simulink model "rocket_model"  (R2012b)
settings: Solver=ode3  StartTime=0.0  StopTime=100  MaxStep=.01  RelTol=1e-3
values from neighbouring files (symbols this model uses):
  coef_body = [0; 0; 0; 0; 0; 0]    [rocket_model_matlab.m]
  cp = [1.2; 0; 0]    [rocket_model_matlab.m]
  dyear = decyear('13-January-2014','dd-mmm-yyyy')    [rocket_model_matlab.m]
  href = 0    [rocket_model_matlab.m]
  lat = 37.4292    [rocket_model_matlab.m]
  lon = -122.1381    [rocket_model_matlab.m]
  phi0 = .1    (= 0.1)    [rocket_model_matlab.m]
  psi0 = -0.3    [rocket_model_matlab.m]
  theta0 = pi/2+.2    (= 1.77079632679)    [rocket_model_matlab.m]
  threshold = 0    [rocket_model_matlab.m]
  Thruster_Moment = r*Thruster_Thrust    (= 0.05)    [rocket_model_matlab.m]
  Thruster_Thrust = 1    [rocket_model_matlab.m]
undefined symbols (not defined in the file or in its folder): Earth, WGS84
libraries: aerolibgravity2 x2, aerolibtransform2 x2, aerolibbdyn x2, aerolibutil x2, aerolibanim x1, aerolibadyn x1, aerolibasang x1, aerolibatmos2 x1, aerolib6dof2 x1, simulink x1
settings Model: Creator=Robbie  LastModifiedBy=Robbie

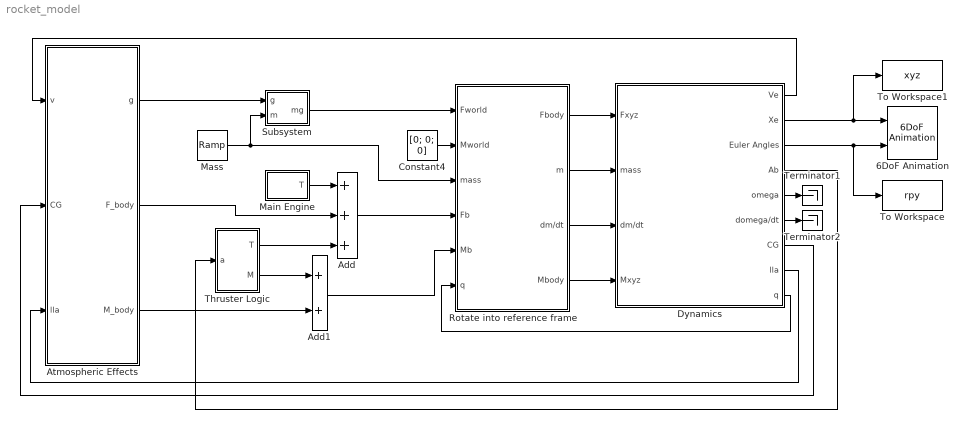
== system rocket_model ==
  6DoF Animation : aerolibanim/6DoF Animation  u1=[0 400 -200 200 -500 -300]  u2=0.1  u3=40  u4=[0 0 40]  u5=Fixed position  u6=[200 50 -315]  u7=10  u8=on
  Add : Sum  Inputs=+++
  Add1 : Sum
  Atmospheric Effects : Subsystem
  Constant4 : Constant  Value=[0; 0; 0]
  Dynamics : Subsystem
  Main Engine : Subsystem
  Mass : simulink/Sources/Ramp  slope=-.2  start=0  X0=50
  Rotate into reference frame : Subsystem
  Subsystem : Subsystem
  Terminator1 : Terminator
  Terminator2 : Terminator
  Thruster Logic : Subsystem
  To Workspace : ToWorkspace  VariableName=rpy  SampleTime=-1  SaveFormat=Timeseries
  To Workspace1 : ToWorkspace  VariableName=xyz  SampleTime=-1  SaveFormat=Timeseries
  wires:
  Dynamics/7(CG) -> Atmospheric Effects/2(CG)
  Dynamics/2(Xe) -> 6DoF Animation/1, To Workspace1/1
  Dynamics/3(Euler Angles) -> 6DoF Animation/2, To Workspace/1
  Dynamics/1(Ve) -> Atmospheric Effects/1(v)
  Dynamics/8(lla) -> Atmospheric Effects/3(lla)
  Atmospheric Effects/3(M_body) -> Add1/2
  Rotate into reference frame/1(Fbody) -> Dynamics/1(Fxyz)
  Rotate into reference frame/4(Mbody) -> Dynamics/4(Mxyz)
  Rotate into reference frame/3(dm/dt) -> Dynamics/3(dm/dt)
  Rotate into reference frame/2(m) -> Dynamics/2(mass)
  Mass/1 -> Subsystem/2(m), Rotate into reference frame/3(mass)
  Atmospheric Effects/2(F_body) -> Add/2
  Main Engine/1(T) -> Add/1
  Dynamics/9(q) -> Rotate into reference frame/6(q)
  Subsystem/1(mg) -> Rotate into reference frame/1(Fworld)
  Add1/1 -> Rotate into reference frame/5(Mb)
  Dynamics/5(omega) -> Terminator1/1
  Dynamics/6(domega/dt) -> Terminator2/1
  Thruster Logic/1(T) -> Add/3
  Thruster Logic/2(M) -> Add1/1
  Constant4/1 -> Rotate into reference frame/2(Mworld)
  Atmospheric Effects/1(g) -> Subsystem/1(g)
  Add/1 -> Rotate into reference frame/4(Fb)
  Dynamics/4(Ab) -> Thruster Logic/1(a)

== system rocket_model/Atmospheric Effects ==
  v : Inport
  CG : Inport  Port=2
  lla : Inport  Port=3
  Aerodynamics Forces : Subsystem
  LLA to Flat Earth (NED) + Atmospheric Model : Subsystem
  g : Outport
  F_body : Outport  Port=2
  M_body : Outport  Port=3
  wires:
  lla/1 -> LLA to Flat Earth (NED) + Atmospheric Model/1(lla)
  LLA to Flat Earth (NED) + Atmospheric Model/2("g (m/s^2) ") -> g/1
  Aerodynamics Forces/1(F_body) -> F_body/1
  v/1 -> Aerodynamics Forces/1(V)
  LLA to Flat Earth (NED) + Atmospheric Model/1(rho (kg/m^3)) -> Aerodynamics Forces/3(rho)
  Aerodynamics Forces/2(M_body) -> M_body/1
  CG/1 -> Aerodynamics Forces/2(CG)

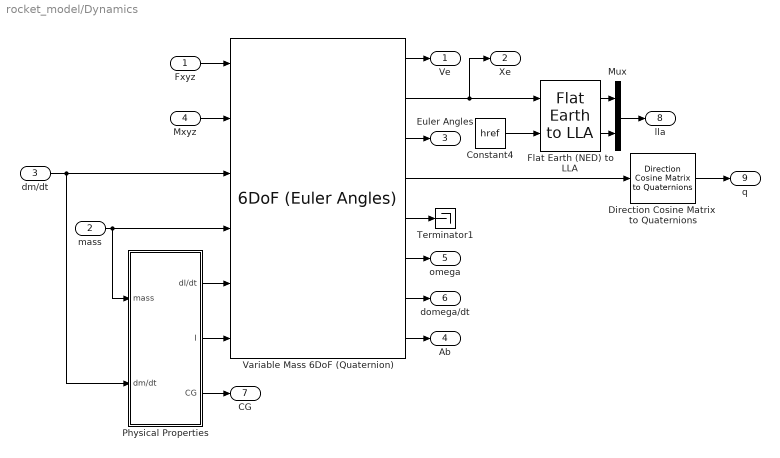
== system rocket_model/Dynamics ==
  Fxyz : Inport
  mass : Inport  Port=2
  dm/dt : Inport  Port=3
  Mxyz : Inport  Port=4
  Constant4 : Constant  Value=href
  Direction Cosine Matrix  to Quaternions : aerolibtransform2/Direction Cosine Matrix  to Quaternions
  Flat Earth (NED) to LLA : aerolibtransform2/Flat Earth to LLA  units=Metric (MKS)  ptype=Earth (WGS84)  F=1/298.257223563  R=6378137  LL0=[lat lon]  psi=0
  Mux : Mux  Inputs=2
  Physical Properties : Subsystem
  Terminator1 : Terminator
  Variable Mass 6DoF (Quaternion) : aerolib6dof2/6DoF (Euler Angles)  units=Metric (MKS)  mtype=Custom Variable  rep=Quaternion  xme_0=[0 0 0]  Vm_0=[0 0 0]  eul_0=[phi0 theta0 psi0]  pm_0=[0 0 0]  mass_0=1.0  mass_e=0  mass_f=0  inertia=eye(3)  inertia_e=eye(3)  inertia_f=eye(3)  k_quat=1.0
  Ve : Outport
  Xe : Outport  Port=2
  Euler Angles : Outport  Port=3
  Ab : Outport  Port=4
  omega : Outport  Port=5
  domega/dt : Outport  Port=6
  CG : Outport  Port=7
  lla : Outport  Port=8
  q : Outport  Port=9
  wires:
  Variable Mass 6DoF (Quaternion)/3 -> Euler Angles/1
  Variable Mass 6DoF (Quaternion)/2 -> Flat Earth (NED) to LLA/1, Xe/1
  Constant4/1 -> Flat Earth (NED) to LLA/2
  Variable Mass 6DoF (Quaternion)/8 -> Ab/1
  dm/dt/1 -> Variable Mass 6DoF (Quaternion)/3, Physical Properties/2(dm/dt)
  Physical Properties/3(CG) -> CG/1
  Physical Properties/1(dI/dt) -> Variable Mass 6DoF (Quaternion)/5
  Physical Properties/2(I) -> Variable Mass 6DoF (Quaternion)/6
  Variable Mass 6DoF (Quaternion)/6 -> omega/1
  Fxyz/1 -> Variable Mass 6DoF (Quaternion)/1
  mass/1 -> Variable Mass 6DoF (Quaternion)/4, Physical Properties/1(mass)
  Variable Mass 6DoF (Quaternion)/7 -> domega/dt/1
  Variable Mass 6DoF (Quaternion)/1 -> Ve/1
  Mxyz/1 -> Variable Mass 6DoF (Quaternion)/2
  Variable Mass 6DoF (Quaternion)/4 -> Direction Cosine Matrix  to Quaternions/1
  Variable Mass 6DoF (Quaternion)/5 -> Terminator1/1
  Flat Earth (NED) to LLA/1 -> Mux/1
  Flat Earth (NED) to LLA/2 -> Mux/2
  Mux/1 -> lla/1
  Direction Cosine Matrix  to Quaternions/1 -> q/1

== system rocket_model/Main Engine ==
  Constant1 : Constant  Value=0
  Constant2 : Constant  Value=0
  Constant3 : Constant  Value=450
  Mux : Mux  Inputs=3
  T : Outport
  wires:
  Constant1/1 -> Mux/3
  Constant3/1 -> Mux/1
  Constant2/1 -> Mux/2
  Mux/1 -> T/1

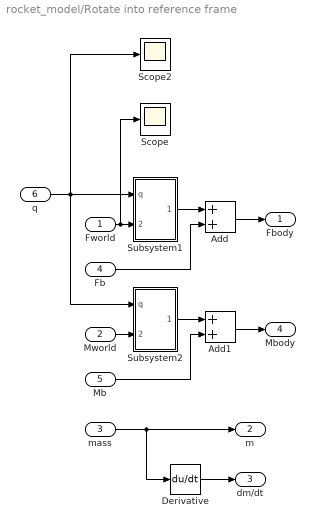
== system rocket_model/Rotate into reference frame ==
  Fworld : Inport
  Mworld : Inport  Port=2
  mass : Inport  Port=3
  Fb : Inport  Port=4
  Mb : Inport  Port=5
  q : Inport  Port=6
  Add : Sum
  Add1 : Sum
  Derivative : Derivative
  Scope : Scope
  Scope2 : Scope
      settings: SaveName=ScopeData2
  Subsystem1 : Subsystem
  Subsystem2 : Subsystem
  Fbody : Outport
  m : Outport  Port=2
  dm/dt : Outport  Port=3
  Mbody : Outport  Port=4
  wires:
  Fworld/1 -> Scope/1, Subsystem1/2(vec)
  Mworld/1 -> Subsystem2/2(vec)
  Subsystem1/1(vec_rot) -> Add/1
  Add/1 -> Fbody/1
  Fb/1 -> Add/2
  Subsystem2/1(vec_rot) -> Add1/1
  Add1/1 -> Mbody/1
  Mb/1 -> Add1/2
  mass/1 -> Derivative/1, m/1
  Derivative/1 -> dm/dt/1
  q/1 -> Scope2/1, Subsystem2/1(q), Subsystem1/1(q)

== system rocket_model/Subsystem ==
  g : Inport
  m : Inport  Port=2
  Product1 : Product  RndMeth=Zero
  mg : Outport
  wires:
  m/1 -> Product1/1
  g/1 -> Product1/2
  Product1/1 -> mg/1

== system rocket_model/Thruster Logic ==
  a : Inport
  Demux : Demux  Outputs=8
  Fire Thruster : Subsystem
  logic : Subsystem
  T : Outport
  M : Outport  Port=2
  wires:
  Demux/7 -> Fire Thruster/7(u7)
  Demux/2 -> Fire Thruster/2(u2)
  Demux/8 -> Fire Thruster/8(u8)
  Demux/6 -> Fire Thruster/6(u6)
  Demux/4 -> Fire Thruster/4(u4)
  Demux/1 -> Fire Thruster/1(u1)
  Demux/5 -> Fire Thruster/5(u5)
  Demux/3 -> Fire Thruster/3(u3)
  Fire Thruster/2(M) -> M/1
  Fire Thruster/1(T) -> T/1
  a/1 -> logic/1("a ")
  logic/1(u) -> Demux/1

== system rocket_model/Atmospheric Effects/Aerodynamics Forces ==
  V : Inport
  CG : Inport  Port=2
  rho : Inport  Port=3
  "Aerodynamic Forces and Moments " : aerolibadyn/Aerodynamic Forces and Moments   inputAxes=Body  outputForceAxes=Body  outputMomentAxes=Body  S=1  b=1  cbar=1
  Constant5 : Constant  Value=cp
  Constant6 : Constant  Value=coef_body
  Dynamic Pressure : aerolibasang/Dynamic Pressure
  F_body : Outport
  M_body : Outport  Port=2
  wires:
  "Aerodynamic Forces and Moments "/2 -> M_body/1
  "Aerodynamic Forces and Moments "/1 -> F_body/1
  Dynamic Pressure/1 -> "Aerodynamic Forces and Moments "/2
  Constant6/1 -> "Aerodynamic Forces and Moments "/1
  Constant5/1 -> "Aerodynamic Forces and Moments "/4
  rho/1 -> Dynamic Pressure/2
  V/1 -> Dynamic Pressure/1
  CG/1 -> "Aerodynamic Forces and Moments "/3

== system rocket_model/Atmospheric Effects/LLA to Flat Earth (NED) + Atmospheric Model ==
  lla : Inport
  Constant1 : Constant  Value=dyear
  Constant4 : Constant  Value=0
  Demux1 : Demux  Outputs=3
  ISA Atmosphere Model : aerolibatmos2/ISA Atmosphere Model  custom=off  g=9.80665  gamma=1.4  R=287.0531  L=0.0065  h_trop=11000  h_strat=20000  rho0=1.225  P0=101325  T0=288.15
  Terminator{1..4} (4 alike) : Terminator
  "WGS84 Gravity Model " : aerolibgravity2/WGS84 Gravity Model   model=WGS84 Taylor Series  units=Metric (MKS)  no_atmos=on  precessing=on  jd_loc=off  month=October  day=10  year=2004  no_centrifugal=on  action=Warning
  World Magnetic Model 2010 : aerolibgravity2/World Magnetic Model 2010  units=Metric (MKS)  time_in=on  month=June  day=12  year=2014  action=Error  h_out=off  dec_out=off  inc_out=off  ti_out=off
  rho (kg/m^3) : Outport
  "g (m/s^2) " : Outport  Port=2
  wires:
  "WGS84 Gravity Model "/1 -> "g (m/s^2) "/1
  ISA Atmosphere Model/1 -> Terminator1/1
  ISA Atmosphere Model/2 -> Terminator2/1
  ISA Atmosphere Model/4 -> rho (kg/m^3)/1
  Constant1/1 -> World Magnetic Model 2010/4
  World Magnetic Model 2010/1 -> Terminator4/1
  ISA Atmosphere Model/3 -> Terminator3/1
  Demux1/3 -> ISA Atmosphere Model/1
  lla/1 -> Demux1/1, "WGS84 Gravity Model "/1
  Demux1/2 -> World Magnetic Model 2010/3
  Demux1/1 -> World Magnetic Model 2010/2
  Constant4/1 -> World Magnetic Model 2010/1

== system rocket_model/Dynamics/Physical Properties ==
  mass : Inport
  dm/dt : Inport  Port=2
  Estimate Center of Gravity : aerolibbdyn/Estimate Center of Gravity  fmass=full_mass  emass=empty_mass  fcg=full_cg  ecg=empty_cg
  Estimate Inertia Tensor : aerolibbdyn/Estimate Inertia Tensor  fmass=full_mass  emass=empty_mass  fI=full_intertia_matrix  eI=empty_intertia_matrix
  Terminator1 : Terminator
  dI/dt : Outport
  I : Outport  Port=2
  CG : Outport  Port=3
  wires:
  Estimate Center of Gravity/2 -> Terminator1/1
  Estimate Inertia Tensor/1 -> I/1
  Estimate Center of Gravity/1 -> CG/1
  Estimate Inertia Tensor/2 -> dI/dt/1
  mass/1 -> Estimate Inertia Tensor/1, Estimate Center of Gravity/1
  dm/dt/1 -> Estimate Inertia Tensor/2, Estimate Center of Gravity/2

== system rocket_model/Rotate into reference frame/Subsystem1 ==
  q : Inport
  vec : Inport  Port=2
  Quaternion Rotation : aerolibutil/Quaternion Rotation
  vec_rot : Outport
  wires:
  vec/1 -> Quaternion Rotation/2
  q/1 -> Quaternion Rotation/1
  Quaternion Rotation/1 -> vec_rot/1

== system rocket_model/Rotate into reference frame/Subsystem2 ==
  q : Inport
  vec : Inport  Port=2
  Quaternion Rotation : aerolibutil/Quaternion Rotation
  vec_rot : Outport
  wires:
  vec/1 -> Quaternion Rotation/2
  q/1 -> Quaternion Rotation/1
  Quaternion Rotation/1 -> vec_rot/1

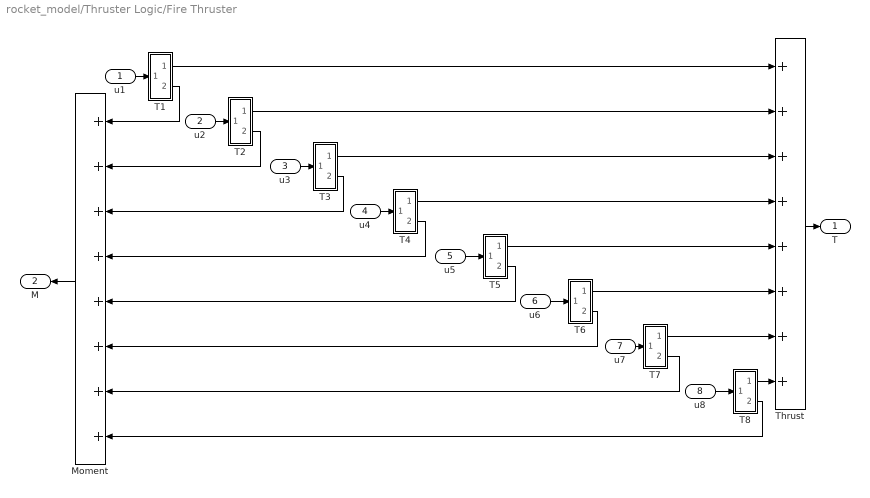
== system rocket_model/Thruster Logic/Fire Thruster ==
  u1 : Inport
  u2 : Inport  Port=2
  u3 : Inport  Port=3
  u4 : Inport  Port=4
  u5 : Inport  Port=5
  u6 : Inport  Port=6
  u7 : Inport  Port=7
  u8 : Inport  Port=8
  Moment : Sum  Inputs=++++++++
  T1 : Subsystem
  T2 : Subsystem
  T3 : Subsystem
  T4 : Subsystem
  T5 : Subsystem
  T6 : Subsystem
  T7 : Subsystem
  T8 : Subsystem
  Thrust : Sum  Inputs=++++++++
  T : Outport
  M : Outport  Port=2
  wires:
  T1/1(T) -> Thrust/1
  T2/1(T) -> Thrust/2
  T3/1(T1) -> Thrust/3
  T1/2(M) -> Moment/1
  T2/2(M) -> Moment/2
  T3/2(M1) -> Moment/3
  T4/1(T) -> Thrust/4
  T5/1(T) -> Thrust/5
  T6/1(T) -> Thrust/6
  T7/1(T) -> Thrust/7
  T8/1(T) -> Thrust/8
  T4/2(M) -> Moment/4
  T5/2(M) -> Moment/5
  T6/2(M) -> Moment/6
  T7/2(M) -> Moment/7
  T8/2(M) -> Moment/8
  u1/1 -> T1/1(u)
  u2/1 -> T2/1(u)
  u3/1 -> T3/1(u)
  u4/1 -> T4/1(u)
  u5/1 -> T5/1(u)
  u6/1 -> T6/1(u)
  u7/1 -> T7/1(u)
  u8/1 -> T8/1(u)
  Thrust/1 -> T/1
  Moment/1 -> M/1

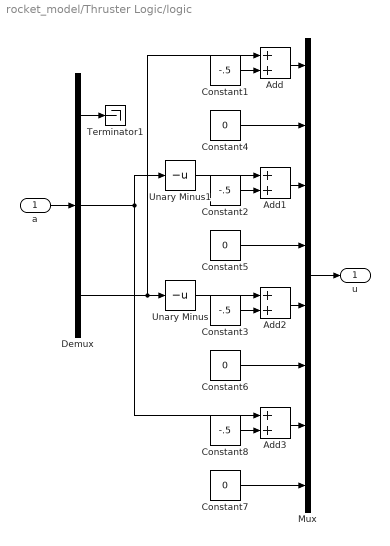
== system rocket_model/Thruster Logic/logic ==
  "a " : Inport
  Add{,1..3} (4 alike) : Sum
  Constant{1..3,8} (4 alike) : Constant  Value=-.5
  Constant{4..7} (4 alike) : Constant  Value=0
  Demux : Demux  Outputs=3
  Mux : Mux  Inputs=8
  Terminator1 : Terminator
  Unary Minus : UnaryMinus
  Unary Minus1 : UnaryMinus
  u : Outport
  wires:
  Demux/3 -> Add/1, Unary Minus/1
  Mux/1 -> u/1
  "a "/1 -> Demux/1
  Demux/2 -> Add3/1, Unary Minus1/1
  Demux/1 -> Terminator1/1
  Constant4/1 -> Mux/2
  Constant7/1 -> Mux/8
  Constant6/1 -> Mux/6
  Constant5/1 -> Mux/4
  Unary Minus1/1 -> Add1/1
  Add2/1 -> Mux/5
  Add1/1 -> Mux/3
  Unary Minus/1 -> Add2/1
  Add3/1 -> Mux/7
  Constant1/1 -> Add/2
  Add/1 -> Mux/1
  Constant2/1 -> Add1/2
  Constant3/1 -> Add2/2
  Constant8/1 -> Add3/2

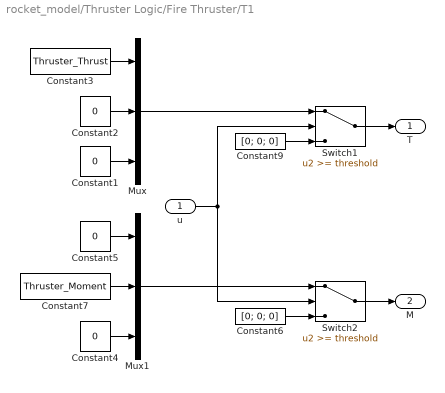
== system rocket_model/Thruster Logic/Fire Thruster/T1 ==
  u : Inport
  Constant{1..2,4..5} (4 alike) : Constant  Value=0
  Constant3 : Constant  Value=Thruster_Thrust
  Constant6 : Constant  Value=[0; 0; 0]
  Constant7 : Constant  Value=Thruster_Moment
  Constant9 : Constant  Value=[0; 0; 0]
  Mux : Mux  Inputs=3
  Mux1 : Mux  Inputs=3
  Switch1 : Switch  Threshold=threshold
  Switch2 : Switch  Threshold=threshold
  T : Outport
  M : Outport  Port=2
  wires:
  Constant1/1 -> Mux/3
  Constant3/1 -> Mux/1
  Constant2/1 -> Mux/2
  Constant4/1 -> Mux1/3
  Constant5/1 -> Mux1/1
  Constant7/1 -> Mux1/2
  Switch1/1 -> T/1
  Mux/1 -> Switch1/1
  Constant9/1 -> Switch1/3
  Switch2/1 -> M/1
  u/1 -> Switch2/2, Switch1/2
  Mux1/1 -> Switch2/1
  Constant6/1 -> Switch2/3

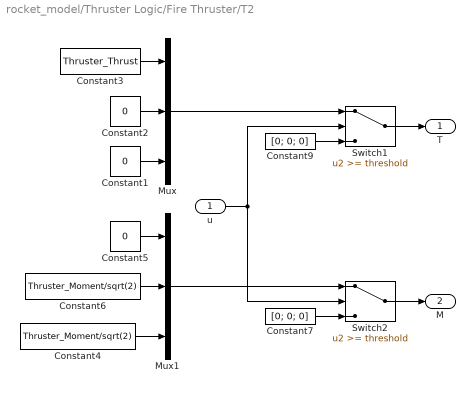
== system rocket_model/Thruster Logic/Fire Thruster/T2 ==
  u : Inport
  Constant1 : Constant  Value=0
  Constant2 : Constant  Value=0
  Constant3 : Constant  Value=Thruster_Thrust
  Constant4 : Constant  Value=Thruster_Moment/sqrt(2)
  Constant5 : Constant  Value=0
  Constant6 : Constant  Value=Thruster_Moment/sqrt(2)
  Constant7 : Constant  Value=[0; 0; 0]
  Constant9 : Constant  Value=[0; 0; 0]
  Mux : Mux  Inputs=3
  Mux1 : Mux  Inputs=3
  Switch1 : Switch  Threshold=threshold
  Switch2 : Switch  Threshold=threshold
  T : Outport
  M : Outport  Port=2
  wires:
  Constant1/1 -> Mux/3
  Constant3/1 -> Mux/1
  Constant2/1 -> Mux/2
  Constant4/1 -> Mux1/3
  Constant5/1 -> Mux1/1
  Constant6/1 -> Mux1/2
  Switch1/1 -> T/1
  Mux/1 -> Switch1/1
  Constant9/1 -> Switch1/3
  Switch2/1 -> M/1
  u/1 -> Switch2/2, Switch1/2
  Mux1/1 -> Switch2/1
  Constant7/1 -> Switch2/3

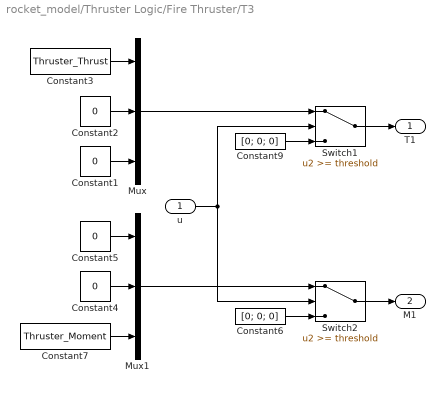
== system rocket_model/Thruster Logic/Fire Thruster/T3 ==
  u : Inport
  Constant{1..2,4..5} (4 alike) : Constant  Value=0
  Constant3 : Constant  Value=Thruster_Thrust
  Constant6 : Constant  Value=[0; 0; 0]
  Constant7 : Constant  Value=Thruster_Moment
  Constant9 : Constant  Value=[0; 0; 0]
  Mux : Mux  Inputs=3
  Mux1 : Mux  Inputs=3
  Switch1 : Switch  Threshold=threshold
  Switch2 : Switch  Threshold=threshold
  T1 : Outport
  M1 : Outport  Port=2
  wires:
  Constant1/1 -> Mux/3
  Constant3/1 -> Mux/1
  Constant2/1 -> Mux/2
  Constant7/1 -> Mux1/3
  Constant5/1 -> Mux1/1
  Constant4/1 -> Mux1/2
  Switch1/1 -> T1/1
  Mux/1 -> Switch1/1
  Constant9/1 -> Switch1/3
  Switch2/1 -> M1/1
  u/1 -> Switch2/2, Switch1/2
  Mux1/1 -> Switch2/1
  Constant6/1 -> Switch2/3

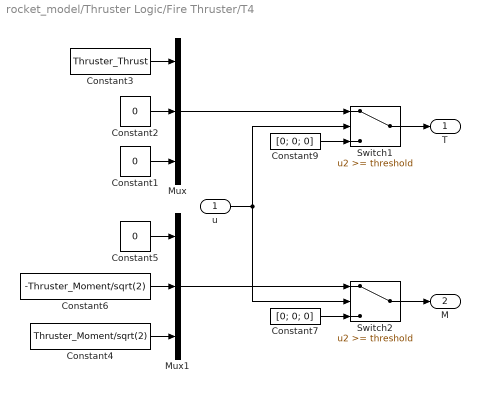
== system rocket_model/Thruster Logic/Fire Thruster/T4 ==
  u : Inport
  Constant1 : Constant  Value=0
  Constant2 : Constant  Value=0
  Constant3 : Constant  Value=Thruster_Thrust
  Constant4 : Constant  Value=Thruster_Moment/sqrt(2)
  Constant5 : Constant  Value=0
  Constant6 : Constant  Value=-Thruster_Moment/sqrt(2)
  Constant7 : Constant  Value=[0; 0; 0]
  Constant9 : Constant  Value=[0; 0; 0]
  Mux : Mux  Inputs=3
  Mux1 : Mux  Inputs=3
  Switch1 : Switch  Threshold=threshold
  Switch2 : Switch  Threshold=threshold
  T : Outport
  M : Outport  Port=2
  wires:
  Constant1/1 -> Mux/3
  Constant3/1 -> Mux/1
  Constant2/1 -> Mux/2
  Constant4/1 -> Mux1/3
  Constant5/1 -> Mux1/1
  Constant6/1 -> Mux1/2
  Switch1/1 -> T/1
  Mux/1 -> Switch1/1
  Constant9/1 -> Switch1/3
  Switch2/1 -> M/1
  u/1 -> Switch2/2, Switch1/2
  Mux1/1 -> Switch2/1
  Constant7/1 -> Switch2/3

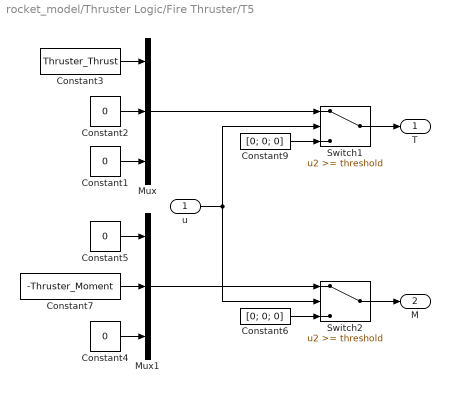
== system rocket_model/Thruster Logic/Fire Thruster/T5 ==
  u : Inport
  Constant{1..2,4..5} (4 alike) : Constant  Value=0
  Constant3 : Constant  Value=Thruster_Thrust
  Constant6 : Constant  Value=[0; 0; 0]
  Constant7 : Constant  Value=-Thruster_Moment
  Constant9 : Constant  Value=[0; 0; 0]
  Mux : Mux  Inputs=3
  Mux1 : Mux  Inputs=3
  Switch1 : Switch  Threshold=threshold
  Switch2 : Switch  Threshold=threshold
  T : Outport
  M : Outport  Port=2
  wires:
  Constant1/1 -> Mux/3
  Constant3/1 -> Mux/1
  Constant2/1 -> Mux/2
  Constant4/1 -> Mux1/3
  Constant5/1 -> Mux1/1
  Constant7/1 -> Mux1/2
  Switch1/1 -> T/1
  Mux/1 -> Switch1/1
  Constant9/1 -> Switch1/3
  Switch2/1 -> M/1
  u/1 -> Switch2/2, Switch1/2
  Mux1/1 -> Switch2/1
  Constant6/1 -> Switch2/3

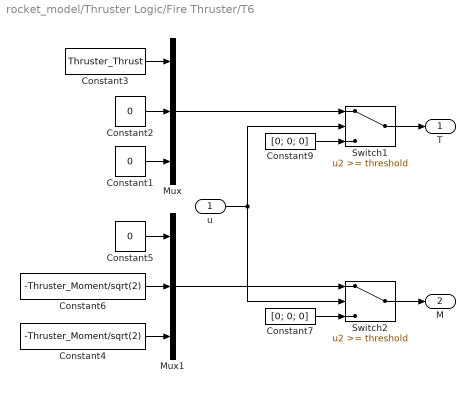
== system rocket_model/Thruster Logic/Fire Thruster/T6 ==
  u : Inport
  Constant1 : Constant  Value=0
  Constant2 : Constant  Value=0
  Constant3 : Constant  Value=Thruster_Thrust
  Constant4 : Constant  Value=-Thruster_Moment/sqrt(2)
  Constant5 : Constant  Value=0
  Constant6 : Constant  Value=-Thruster_Moment/sqrt(2)
  Constant7 : Constant  Value=[0; 0; 0]
  Constant9 : Constant  Value=[0; 0; 0]
  Mux : Mux  Inputs=3
  Mux1 : Mux  Inputs=3
  Switch1 : Switch  Threshold=threshold
  Switch2 : Switch  Threshold=threshold
  T : Outport
  M : Outport  Port=2
  wires:
  Constant1/1 -> Mux/3
  Constant3/1 -> Mux/1
  Constant2/1 -> Mux/2
  Constant4/1 -> Mux1/3
  Constant5/1 -> Mux1/1
  Constant6/1 -> Mux1/2
  Switch1/1 -> T/1
  Mux/1 -> Switch1/1
  Constant9/1 -> Switch1/3
  Switch2/1 -> M/1
  u/1 -> Switch2/2, Switch1/2
  Mux1/1 -> Switch2/1
  Constant7/1 -> Switch2/3

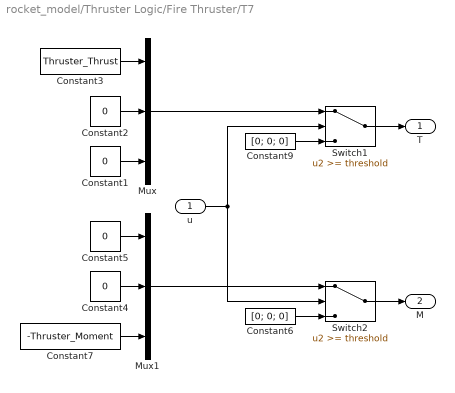
== system rocket_model/Thruster Logic/Fire Thruster/T7 ==
  u : Inport
  Constant{1..2,4..5} (4 alike) : Constant  Value=0
  Constant3 : Constant  Value=Thruster_Thrust
  Constant6 : Constant  Value=[0; 0; 0]
  Constant7 : Constant  Value=-Thruster_Moment
  Constant9 : Constant  Value=[0; 0; 0]
  Mux : Mux  Inputs=3
  Mux1 : Mux  Inputs=3
  Switch1 : Switch  Threshold=threshold
  Switch2 : Switch  Threshold=threshold
  T : Outport
  M : Outport  Port=2
  wires:
  Constant1/1 -> Mux/3
  Constant3/1 -> Mux/1
  Constant2/1 -> Mux/2
  Constant7/1 -> Mux1/3
  Constant5/1 -> Mux1/1
  Constant4/1 -> Mux1/2
  Switch1/1 -> T/1
  Mux/1 -> Switch1/1
  Constant9/1 -> Switch1/3
  Switch2/1 -> M/1
  u/1 -> Switch2/2, Switch1/2
  Mux1/1 -> Switch2/1
  Constant6/1 -> Switch2/3

== system rocket_model/Thruster Logic/Fire Thruster/T8 ==
  u : Inport
  Constant1 : Constant  Value=0
  Constant2 : Constant  Value=0
  Constant3 : Constant  Value=Thruster_Thrust
  Constant4 : Constant  Value=Thruster_Moment/sqrt(2)
  Constant5 : Constant  Value=0
  Constant6 : Constant  Value=-Thruster_Moment/sqrt(2)
  Constant7 : Constant  Value=[0; 0; 0]
  Constant9 : Constant  Value=[0; 0; 0]
  Mux : Mux  Inputs=3
  Mux1 : Mux  Inputs=3
  Switch1 : Switch  Threshold=threshold
  Switch2 : Switch  Threshold=threshold
  T : Outport
  M : Outport  Port=2
  wires:
  Constant1/1 -> Mux/3
  Constant3/1 -> Mux/1
  Constant2/1 -> Mux/2
  Constant6/1 -> Mux1/3
  Constant5/1 -> Mux1/1
  Constant4/1 -> Mux1/2
  Switch1/1 -> T/1
  Mux/1 -> Switch1/1
  Constant9/1 -> Switch1/3
  Switch2/1 -> M/1
  u/1 -> Switch2/2, Switch1/2
  Mux1/1 -> Switch2/1
  Constant7/1 -> Switch2/3
